simulink model "Exp_3_batch_12_simulation5"  (R2020a)
settings: Solver=VariableStepAuto  StartTime=0.0  StopTime=20  RelTol=1e-3
settings Model: Creator=sundaram bhupathi  LastModifiedBy=sundaram bhupathi

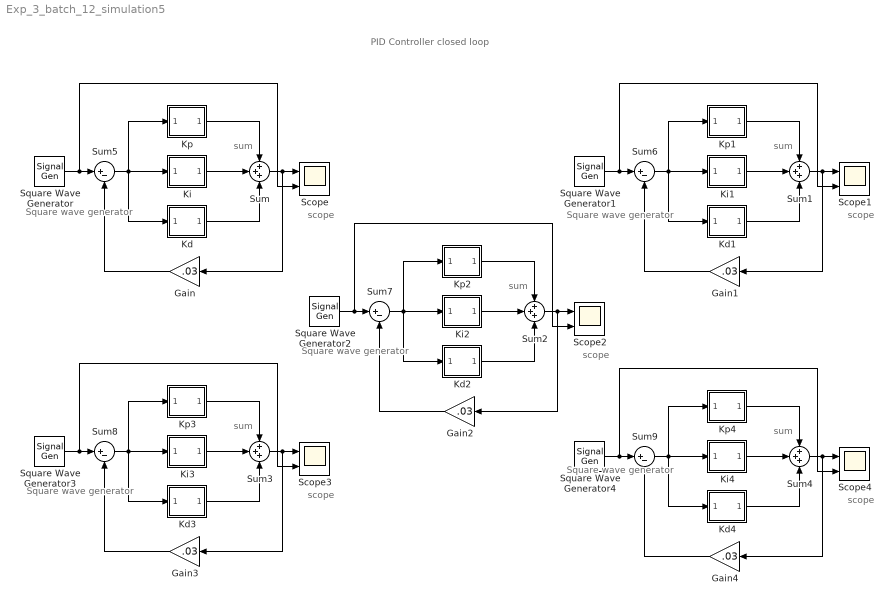
== system Exp_3_batch_12_simulation5 ==
  note: PID Controller closed loop
  note: sum
  note: scope
  note: Square wave generator
  note: scope
  note: Square wave generator
  note: sum
  note: scope
  note: Square wave generator
  note: sum
  note: scope
  note: Square wave generator
  note: sum
  note: scope
  note: Square wave generator
  note: sum
  Gain{,1..4} (5 alike) : Gain  Gain=.03
  Kd : Subsystem
  Kd1 : Subsystem
  Kd2 : Subsystem
  Kd3 : Subsystem
  Kd4 : Subsystem
  Ki : Subsystem
  Ki1 : Subsystem
  Ki2 : Subsystem
  Ki3 : Subsystem
  Ki4 : Subsystem
  Kp : Subsystem
  Kp1 : Subsystem
  Kp2 : Subsystem
  Kp3 : Subsystem
  Kp4 : Subsystem
  Scope{,1..4} (5 alike) : Scope  NumInputPorts=2
  Square Wave Generator{,1..4} (5 alike) : SignalGenerator  WaveForm=square  Amplitude=10  Units=rad/sec
  Sum{,1..4} (5 alike) : Sum  Inputs=+++  InputSameDT=on  SaturateOnIntegerOverflow=on  OutDataTypeStr=Inherit: Same as first input
  Sum{5..9} (5 alike) : Sum  Inputs=|+-
  wires:
  Kd/1(Out1) -> Sum/3
  Kp/1(Out1) -> Sum/1
  Ki/1(Out1) -> Sum/2
  Sum/1 -> Gain/1, Scope/1
  Square Wave Generator/1 -> Scope/2, Sum5/1
  Sum5/1 -> Kd/1(In1), Kp/1(In1), Ki/1(In1)
  Gain/1 -> Sum5/2
  Ki1/1(Out1) -> Sum1/2
  Square Wave Generator1/1 -> Scope1/2, Sum6/1
  Sum1/1 -> Gain1/1, Scope1/1
  Kd1/1(Out1) -> Sum1/3
  Kp1/1(Out1) -> Sum1/1
  Gain1/1 -> Sum6/2
  Sum6/1 -> Kd1/1(In1), Kp1/1(In1), Ki1/1(In1)
  Ki2/1(Out1) -> Sum2/2
  Square Wave Generator2/1 -> Scope2/2, Sum7/1
  Sum2/1 -> Gain2/1, Scope2/1
  Kd2/1(Out1) -> Sum2/3
  Kp2/1(Out1) -> Sum2/1
  Gain2/1 -> Sum7/2
  Sum7/1 -> Kd2/1(In1), Kp2/1(In1), Ki2/1(In1)
  Ki3/1(Out1) -> Sum3/2
  Square Wave Generator3/1 -> Scope3/2, Sum8/1
  Sum3/1 -> Gain3/1, Scope3/1
  Kd3/1(Out1) -> Sum3/3
  Kp3/1(Out1) -> Sum3/1
  Gain3/1 -> Sum8/2
  Sum8/1 -> Kd3/1(In1), Kp3/1(In1), Ki3/1(In1)
  Ki4/1(Out1) -> Sum4/2
  Square Wave Generator4/1 -> Scope4/2, Sum9/1
  Sum4/1 -> Gain4/1, Scope4/1
  Kd4/1(Out1) -> Sum4/3
  Kp4/1(Out1) -> Sum4/1
  Gain4/1 -> Sum9/2
  Sum9/1 -> Kd4/1(In1), Kp4/1(In1), Ki4/1(In1)

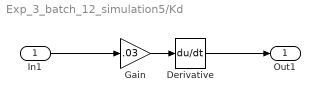
== system Exp_3_batch_12_simulation5/Kd ==
  In1 : Inport
  Derivative : Derivative
  Gain : Gain  Gain=.03
  Out1 : Outport
  wires:
  In1/1 -> Gain/1
  Gain/1 -> Derivative/1
  Derivative/1 -> Out1/1

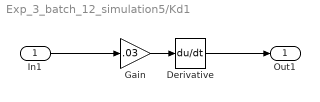
== system Exp_3_batch_12_simulation5/Kd1 ==
  In1 : Inport
  Derivative : Derivative
  Gain : Gain  Gain=.03
  Out1 : Outport
  wires:
  In1/1 -> Gain/1
  Gain/1 -> Derivative/1
  Derivative/1 -> Out1/1

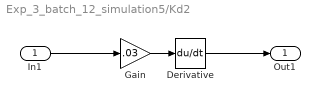
== system Exp_3_batch_12_simulation5/Kd2 ==
  In1 : Inport
  Derivative : Derivative
  Gain : Gain  Gain=.03
  Out1 : Outport
  wires:
  In1/1 -> Gain/1
  Gain/1 -> Derivative/1
  Derivative/1 -> Out1/1

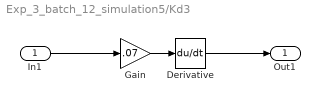
== system Exp_3_batch_12_simulation5/Kd3 ==
  In1 : Inport
  Derivative : Derivative
  Gain : Gain  Gain=.07
  Out1 : Outport
  wires:
  In1/1 -> Gain/1
  Gain/1 -> Derivative/1
  Derivative/1 -> Out1/1

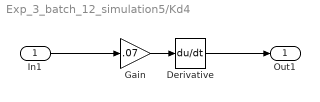
== system Exp_3_batch_12_simulation5/Kd4 ==
  In1 : Inport
  Derivative : Derivative
  Gain : Gain  Gain=.07
  Out1 : Outport
  wires:
  In1/1 -> Gain/1
  Gain/1 -> Derivative/1
  Derivative/1 -> Out1/1

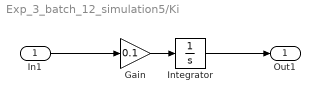
== system Exp_3_batch_12_simulation5/Ki ==
  In1 : Inport
  Gain : Gain  Gain=0.1
  Integrator : Integrator
  Out1 : Outport
  wires:
  In1/1 -> Gain/1
  Gain/1 -> Integrator/1
  Integrator/1 -> Out1/1

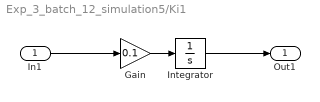
== system Exp_3_batch_12_simulation5/Ki1 ==
  In1 : Inport
  Gain : Gain  Gain=0.1
  Integrator : Integrator
  Out1 : Outport
  wires:
  In1/1 -> Gain/1
  Gain/1 -> Integrator/1
  Integrator/1 -> Out1/1

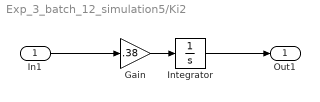
== system Exp_3_batch_12_simulation5/Ki2 ==
  In1 : Inport
  Gain : Gain  Gain=.38
  Integrator : Integrator
  Out1 : Outport
  wires:
  In1/1 -> Gain/1
  Gain/1 -> Integrator/1
  Integrator/1 -> Out1/1

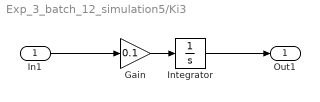
== system Exp_3_batch_12_simulation5/Ki3 ==
  In1 : Inport
  Gain : Gain  Gain=0.1
  Integrator : Integrator
  Out1 : Outport
  wires:
  In1/1 -> Gain/1
  Gain/1 -> Integrator/1
  Integrator/1 -> Out1/1

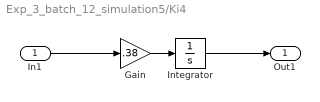
== system Exp_3_batch_12_simulation5/Ki4 ==
  In1 : Inport
  Gain : Gain  Gain=.38
  Integrator : Integrator
  Out1 : Outport
  wires:
  In1/1 -> Gain/1
  Gain/1 -> Integrator/1
  Integrator/1 -> Out1/1

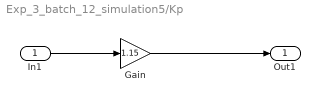
== system Exp_3_batch_12_simulation5/Kp ==
  In1 : Inport
  Gain : Gain  Gain=1.15
  Out1 : Outport
  wires:
  In1/1 -> Gain/1
  Gain/1 -> Out1/1

== system Exp_3_batch_12_simulation5/Kp1 ==
  In1 : Inport
  Gain : Gain  Gain=2
  Out1 : Outport
  wires:
  In1/1 -> Gain/1
  Gain/1 -> Out1/1

== system Exp_3_batch_12_simulation5/Kp2 ==
  In1 : Inport
  Gain : Gain  Gain=1.15
  Out1 : Outport
  wires:
  In1/1 -> Gain/1
  Gain/1 -> Out1/1

== system Exp_3_batch_12_simulation5/Kp3 ==
  In1 : Inport
  Gain : Gain  Gain=1.15
  Out1 : Outport
  wires:
  In1/1 -> Gain/1
  Gain/1 -> Out1/1

== system Exp_3_batch_12_simulation5/Kp4 ==
  In1 : Inport
  Gain : Gain  Gain=2
  Out1 : Outport
  wires:
  In1/1 -> Gain/1
  Gain/1 -> Out1/1
